simulink model "Stimuli"  (R2017b)
settings: Solver=FixedStepAuto  StartTime=0.0  StopTime=10.0  FixedStep=1.0  RelTol=1e-3
settings Model: Creator=eh6qym  LastModifiedBy=eh6qym

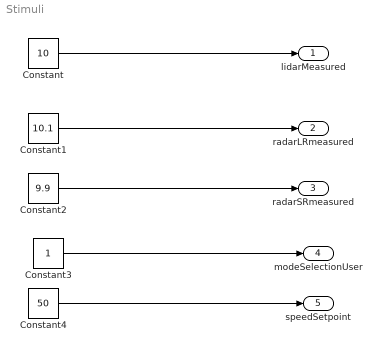
== system Stimuli ==
  Constant : Constant  Value=10  OutDataTypeStr=double
  Constant1 : Constant  Value=10.1  OutDataTypeStr=double
  Constant2 : Constant  Value=9.9  OutDataTypeStr=double
  Constant3 : Constant  OutDataTypeStr=boolean
  Constant4 : Constant  Value=50  OutDataTypeStr=double
  lidarMeasured : Outport  OutDataTypeStr=double  Unit=m
  radarLRmeasured : Outport  Port=2  OutDataTypeStr=double  Unit=m
  radarSRmeasured : Outport  Port=3  OutDataTypeStr=double  Unit=m
  modeSelectionUser : Outport  Port=4  OutDataTypeStr=boolean
  speedSetpoint : Outport  Port=5  OutDataTypeStr=double  Unit=kmh
  wires:
  Constant/1 -> lidarMeasured/1
  Constant1/1 -> radarLRmeasured/1
  Constant2/1 -> radarSRmeasured/1
  Constant3/1 -> modeSelectionUser/1
  Constant4/1 -> speedSetpoint/1
